simulink model "hw4_sim"  (R2016a)
settings: Solver=FixedStepDiscrete  StartTime=0.0  StopTime=86400  FixedStep=1  RelTol=1e-3
values from neighbouring files (symbols this model uses):
  omega = omega /pi*180    (= 0)    [XV2OE.m]
undefined symbols (not defined in the file or in its folder): M0, n0, tOffset, UTC_0
settings Model: Creator=Toby  LastModifiedBy=User
settings DataIOCC: LimitDataPoints=on  SaveFormat=Array
settings HardwareCC: ProdBitPerPointer=32  ProdLargestAtomicFloat=None  ProdIntDivRoundTo=Undefined  ProdEndianess=Unspecified  ProdWordSize=32  ProdHWDeviceType=32-bit Generic
settings ModelReferenceCC: PropagateSignalLabelsOutOfModel=off
settings ConfigComp: CovModelRefEnable=Off

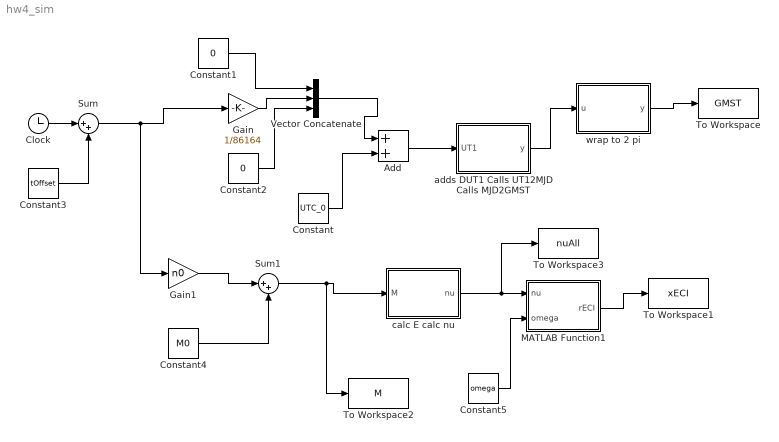
== system hw4_sim ==
  Add : Sum
  Clock : Clock
  Constant : Constant  Value=UTC_0
  Constant1 : Constant  Value=0
  Constant2 : Constant  Value=0
  Constant3 : Constant  Value=tOffset
  Constant4 : Constant  Value=M0
  Constant5 : Constant  Value=omega
  Gain : Gain  Gain=1/86164
  Gain1 : Gain  Gain=n0
  MATLAB Function1 : MATLAB Function  TreatAsAtomicUnit=on
  Sum : Sum  Inputs=|++
  Sum1 : Sum  Inputs=|++
  To Workspace : ToWorkspace  VariableName=GMST  SampleTime=-1
  To Workspace1 : ToWorkspace  VariableName=xECI  SampleTime=-1
  To Workspace2 : ToWorkspace  VariableName=M  SampleTime=-1
  To Workspace3 : ToWorkspace  VariableName=nuAll  SampleTime=-1
  Vector Concatenate : Concatenate  NumInputs=3
  adds DUT1 Calls UT12MJD Calls MJD2GMST : MATLAB Function  TreatAsAtomicUnit=on
  calc E calc nu : MATLAB Function  TreatAsAtomicUnit=on
  wrap to 2 pi : MATLAB Function  TreatAsAtomicUnit=on
  wires:
  Constant/1 -> Add/2
  Clock/1 -> Sum/1
  Constant2/1 -> Vector Concatenate/3
  Gain/1 -> Vector Concatenate/2
  Constant1/1 -> Vector Concatenate/1
  Vector Concatenate/1 -> Add/1
  Add/1 -> adds DUT1 Calls UT12MJD Calls MJD2GMST/1(UT1)
  adds DUT1 Calls UT12MJD Calls MJD2GMST/1(y) -> wrap to 2 pi/1(u)
  Constant3/1 -> Sum/2
  Sum/1 -> Gain1/1, Gain/1
  Constant4/1 -> Sum1/2
  Gain1/1 -> Sum1/1
  Sum1/1 -> To Workspace2/1, calc E calc nu/1(M)
  calc E calc nu/1(nu) -> To Workspace3/1, MATLAB Function1/1(nu)
  MATLAB Function1/1(rECI) -> To Workspace1/1
  wrap to 2 pi/1(y) -> To Workspace/1
  Constant5/1 -> MATLAB Function1/2(omega)

== matlab function hw4_sim/calc E calc nu ==
  data: M input; nu output
function nu = fcn(M)
%M in degrees
e = .6908;
E = calcE(M/180*pi, e, 1e-3); %output in rads
nu = 2*atan2d(sqrt(1+e)*tan(E/2), sqrt(1-e)); %input in rads, output degrees
end

== matlab function hw4_sim/adds DUT1 Calls UT12MJD Calls MJD2GMST ==
  data: UT1 input; y output
function y = fcn(UT1)
%u is calendar form
% DUT1= (UT1-UTC) transmitted with time signals                         
%              =  +0.5 seconds beginning 26 Jan 2017 at 0000 UTC  
UT1(2) = UT1(2) + 0.5/86400; %defined offset
y1 = UT12MJD(UT1);
y = MJD2GMST(y1);
%y in radians
end

== matlab function hw4_sim/MATLAB Function1 ==
  data: nu input; rECI output; omega input
function rECI = fcn(nu, omega)
%#codegen
a = 26521.2313; %km
e = 0.6908;
incl = 64.0353; %all angles in degrees
OMEGA = 80.1299;
rECI = OE2XV(a, e, incl, OMEGA, omega, nu);

== matlab function hw4_sim/wrap to 2 pi ==
  data: u input; y output
function y = fcn(u)
%#codegen

y = wrapTo2Pi(u);
